simulink model "EngineTorqueGeneration"  (R2025b)
settings: Solver=FixedStepAuto  StartTime=0.0  StopTime=10.0  RelTol=1e-3
undefined symbols (not defined in the file): beta0, H_l, k_eta, lambda, nu0, nu1, sigma0, Vd
settings Model: Creator=khanh  LastModifiedBy=khanh

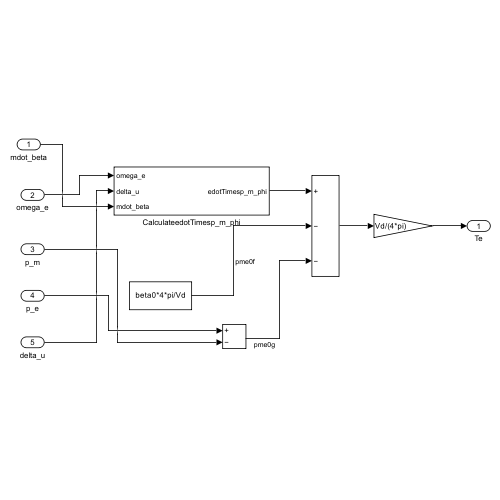
[thumbnail: Simulink's stored preview of the top-level diagram]
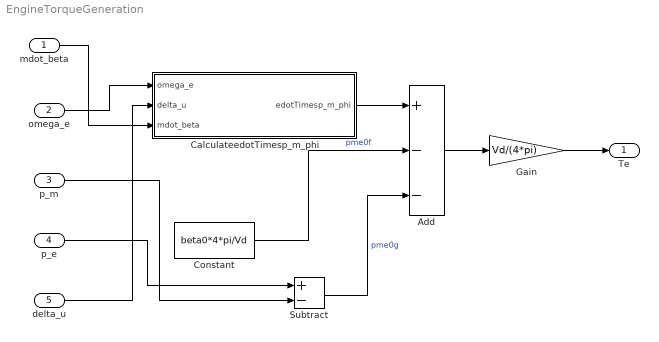
== system EngineTorqueGeneration ==
  mdot_beta : Inport
  omega_e : Inport  Port=2
  p_m : Inport  Port=3
  p_e : Inport  Port=4
  delta_u : Inport  Port=5
  Add : Sum  Inputs=+--
  CalculateedotTimesp_m_phi : Subsystem
  Constant : Constant  Value=beta0*4*pi/Vd
  Gain : Gain  Gain=Vd/(4*pi)
  Subtract : Sum  Inputs=+-
  Te : Outport
  wires:
  omega_e/1 -> CalculateedotTimesp_m_phi/1(omega_e)
  delta_u/1 -> CalculateedotTimesp_m_phi/2(delta_u)
  mdot_beta/1 -> CalculateedotTimesp_m_phi/3(mdot_beta)
  Constant/1 -> Add/2  "pme0f"
  p_e/1 -> Subtract/1
  p_m/1 -> Subtract/2
  Subtract/1 -> Add/3  "pme0g"
  Add/1 -> Gain/1
  Gain/1 -> Te/1
  CalculateedotTimesp_m_phi/1(edotTimesp_m_phi) -> Add/1

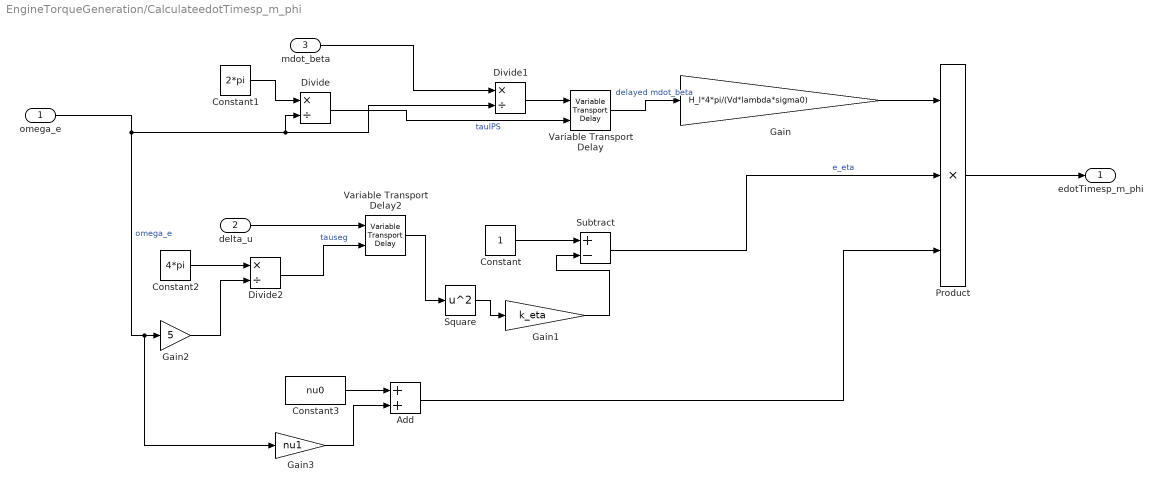
== system EngineTorqueGeneration/CalculateedotTimesp_m_phi ==
  omega_e : Inport
  delta_u : Inport  Port=2
  mdot_beta : Inport  Port=3
  Add : Sum
  Constant : Constant
  Constant1 : Constant  Value=2*pi
  Constant2 : Constant  Value=4*pi
  Constant3 : Constant  Value=nu0
  Divide : Product  Inputs=*/
  Divide1 : Product  Inputs=*/
  Divide2 : Product  Inputs=*/
  Gain : Gain  Gain=H_l*4*pi/(Vd*lambda*sigma0)
  Gain1 : Gain  Gain=k_eta
  Gain2 : Gain  Gain=5
  Gain3 : Gain  Gain=nu1
  Product : Product  Inputs=3
  Square : Math  Operator=square
  Subtract : Sum  Inputs=+-
  Variable Transport Delay : VariableTransportDelay  VariableDelayType=Variable transport delay  MaximumDelay=10
  Variable Transport Delay2 : VariableTransportDelay  VariableDelayType=Variable transport delay  MaximumDelay=10
  edotTimesp_m_phi : Outport
  wires:
  Constant/1 -> Subtract/1
  Gain1/1 -> Subtract/2
  Subtract/1 -> Product/2  "e_eta"
  omega_e/1 -> Gain3/1, Gain2/1, Divide1/2, Divide/2  "omega_e"
  Constant1/1 -> Divide/1
  Constant2/1 -> Divide2/1
  Gain2/1 -> Divide2/2
  Divide2/1 -> Variable Transport Delay2/2  "tauseg"
  delta_u/1 -> Variable Transport Delay2/1
  Constant3/1 -> Add/1
  Gain3/1 -> Add/2
  Gain/1 -> Product/1
  Add/1 -> Product/3
  Product/1 -> edotTimesp_m_phi/1
  Divide/1 -> Variable Transport Delay/2  "tauIPS"
  mdot_beta/1 -> Divide1/1
  Divide1/1 -> Variable Transport Delay/1
  Variable Transport Delay/1 -> Gain/1  "delayed mdot_beta"
  Variable Transport Delay2/1 -> Square/1
  Square/1 -> Gain1/1
